simulink model "joint_impedance_control"  (R2025a)
settings: Solver=FixedStepDiscrete  StartTime=0.0  StopTime=inf  FixedStep=0.001  RelTol=1e-3
PreLoadFcn:
  | frs = FrankaRobotSettings;
libraries: franka_simulink x1
settings Model: SimulationMode=external  ExtModeTrigDuration=10000  Creator=vasi_ko  LastModifiedBy=kvasios
settings SolverCC: ConcurrentTasks=on  AlgebraicLoopSolver=TrustRegion
settings DataIOCC: LimitDataPoints=on  SaveFormat=Array  ReturnWorkspaceOutputs=off
settings OptimizationCC: EnhancedBackFolding=on  PassReuseOutputArgsThreshold=0.0  OptimizeBlockOrder=speed  DifferentSizesBufferReuse=on  OptimizationCustomize=off
settings DebuggingCC: SolverPrmCheckMsg=warning  ParameterTunabilityLossMsg=error  UnconnectedInputMsg=warning  UnconnectedOutputMsg=warning  UnconnectedLineMsg=warning  SFUnexpectedBacktrackingDiag=warning  SFNoUnconditionalDefaultTransitionDiag=warning  SFExecutionAtInitializationDiag=none  ArithmeticOperatorsInVariantConditions=warning
settings HardwareCC: ProdBitPerLong=64.0  ProdHWDeviceType=Intel->x86-64 (Linux 64)
settings ModelReferenceCC: EnableRefExpFcnMdlSchedulingChecks=on  PropagateSignalLabelsOutOfModel=off
settings SFSimCC: SimUseLocalCustomCode=off  MATLABDynamicMemAlloc=off  CustomCodeUndefinedFunction=UseInterfaceOnly  SimTargetLang=C++  SimDLTargetLibrary=mkl-dnn
settings RTWCC: HardwareBoard=Generic Linux AMD64 Board  RTWUseLocalCustomCode=off  BuildConfiguration=Faster Runs  TargetLang=C++  GPUComputeCapability=3.5  DLArmComputeVersion=19.05
settings CodeAppCC: ForceParamTrailComments=on  OperatorAnnotations=on
settings GRTTargetCC: ExtMode=on  ExtModeStaticAlloc=on  ExtModeMexFile=ext_xcp  ExtModeIntrfLevel=Level2 - Open  TargetLangStandard=C++14 (ISO)
settings ConfigComp: CovMetricSettings=dw  CovSaveCumulativeToWorkspaceVar=on  CovSaveSingleToWorkspaceVar=on  CovExternalEMLEnable=off  CovSFcnEnable=off

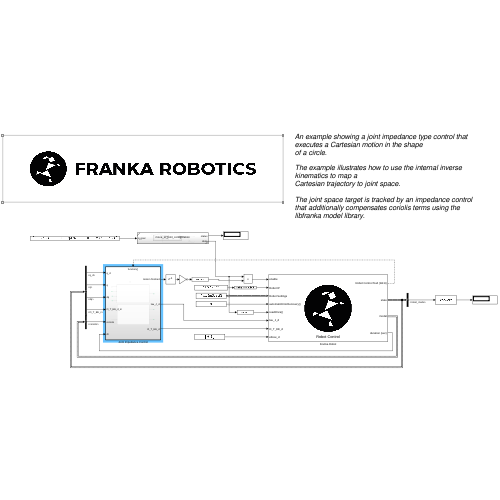
[thumbnail: Simulink's stored preview of the top-level diagram]
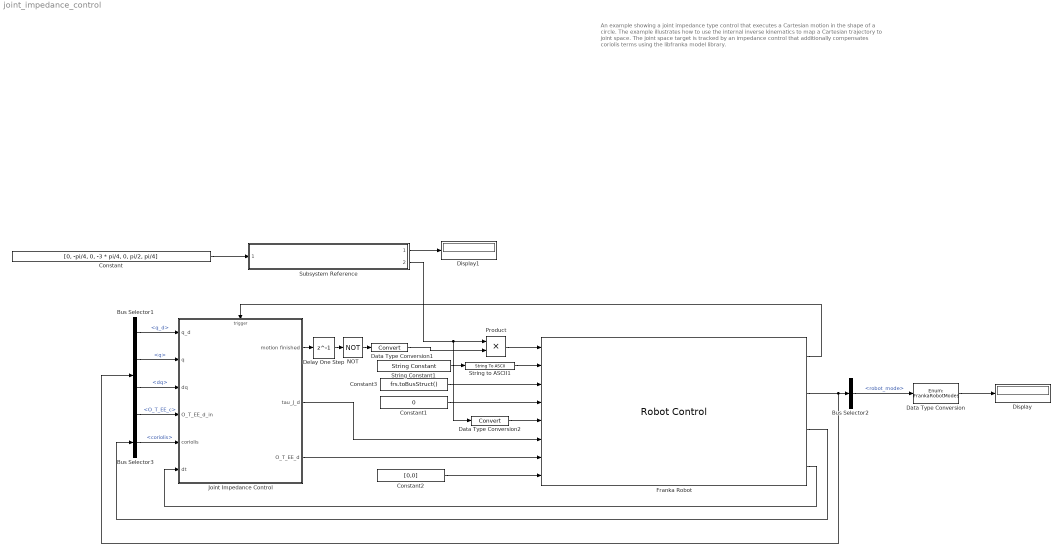
== system joint_impedance_control ==
  note: An example showing a joint impedance type control that executes a Cartesian motion in the shape
      | of a circle.
      |
      | The example illustrates how to use the internal inverse kinematics to map a
      | Cartesian trajectory to joint space.
      |
      | The joint space target is tracked by an impedance control
      | that additionally compensates coriolis terms using the libfranka model library.
  Bus Selector1 : BusSelector  OutputSignals=q_d,q,dq,O_T_EE_c
  Bus Selector2 : BusSelector  OutputSignals=robot_mode
  Bus Selector3 : BusSelector  OutputSignals=coriolis
  Constant : Constant  Value=[0, -pi/4, 0, -3 * pi/4, 0, pi/2, pi/4]
  Constant1 : Constant  Value=0  OutDataTypeStr=Inherit: Inherit via back propagation
  Constant2 : Constant  Value=[0,0]  OutDataTypeStr=Inherit: Inherit via back propagation
  Constant3 : Constant  Value=frs.toBusStruct()  OutDataTypeStr=Bus: FrankaRobotSettingsBus
  Data Type Conversion : DataTypeConversion  OutDataTypeStr=Enum: FrankaRobotModes  SaturateOnIntegerOverflow=off  RndMeth=Floor
  Data Type Conversion1 : DataTypeConversion  SaturateOnIntegerOverflow=off  RndMeth=Floor
  Data Type Conversion2 : DataTypeConversion  SaturateOnIntegerOverflow=off  RndMeth=Floor
  Delay One Step : Delay  DelayLength=1
  Display : Display
  Display1 : Display
  Franka Robot : franka_simulink/Robot Control  control_mode=Torques + Cartesian Pose
      settings: SourceProductName=Franka Robotics Simulink Support Package
  Joint Impedance Control : Subsystem  TreatAsAtomicUnit=on
      settings: RTWSystemCode=Nonreusable function
  NOT : Logic  Operator=NOT  IconShape=distinctive  AllPortsSameDT=off  OutDataTypeStr=boolean
  Product : Product
  String Constant1 : StringConstant  String="\"172.16.0.2\""
  String to ASCII1 : StringToASCII  OutputVectorSize=16
  Subsystem Reference : Subsystem  ReferencedSubsystem=move_to_joint_configuration
  wires:
  Constant/1 -> Subsystem Reference/1
  Bus Selector2/1 -> Data Type Conversion/1  "<robot_mode>"
  Constant3/1 -> Franka Robot/3
  Franka Robot/4 -> Joint Impedance Control/6(dt)
  Joint Impedance Control/1(motion finished) -> Delay One Step/1
  Constant1/1 -> Franka Robot/4
  NOT/1 -> Data Type Conversion1/1
  Data Type Conversion1/1 -> Product/2
  Franka Robot/3 -> Bus Selector3/1
  Subsystem Reference/2 -> Product/1, Data Type Conversion2/1
  Franka Robot/1 -> Joint Impedance Control/Trigger
  Delay One Step/1 -> NOT/1
  Data Type Conversion/1 -> Display/1
  Franka Robot/2 -> Bus Selector1/1, Bus Selector2/1
  String Constant1/1 -> String to ASCII1/1
  Subsystem Reference/1 -> Display1/1
  String to ASCII1/1 -> Franka Robot/2
  Constant2/1 -> Franka Robot/8
  Joint Impedance Control/3(O_T_EE_d) -> Franka Robot/7
  Joint Impedance Control/2(tau_J_d) -> Franka Robot/6
  Bus Selector3/1 -> Joint Impedance Control/5(coriolis)  "<coriolis>"
  Bus Selector1/1 -> Joint Impedance Control/1(q_d)  "<q_d>"
  Bus Selector1/2 -> Joint Impedance Control/2(q)  "<q>"
  Bus Selector1/3 -> Joint Impedance Control/3(dq)  "<dq>"
  Product/1 -> Franka Robot/1
  Data Type Conversion2/1 -> Franka Robot/5
  Bus Selector1/4 -> Joint Impedance Control/4(O_T_EE_d_in)  "<O_T_EE_c>"

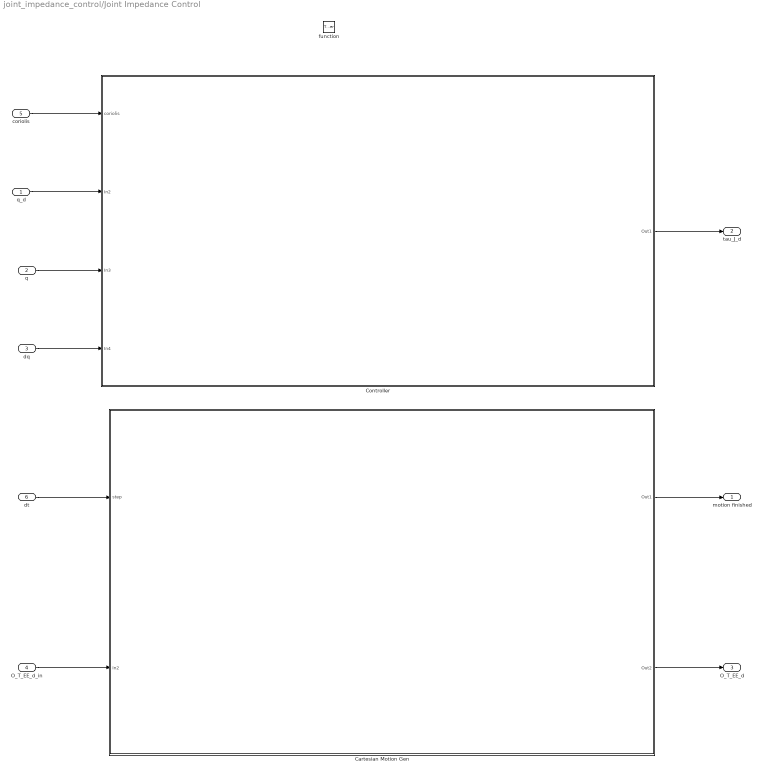
== system joint_impedance_control/Joint Impedance Control ==
  q_d : Inport
  q : Inport  Port=2
  dq : Inport  Port=3
  O_T_EE_d_in : Inport  Port=4
  coriolis : Inport  Port=5
  dt : Inport  Port=6
  function : TriggerPort  TriggerType=function-call  VariantControl=(inherit)
  Cartesian Motion Gen : Subsystem  TreatAsAtomicUnit=on
  Controller : Subsystem  TreatAsAtomicUnit=on
  motion finished : Outport  VectorParamsAs1DForOutWhenUnconnected=off
  tau_J_d : Outport  Port=2  VectorParamsAs1DForOutWhenUnconnected=off
  O_T_EE_d : Outport  Port=3  VectorParamsAs1DForOutWhenUnconnected=off
  wires:
  coriolis/1 -> Controller/1(coriolis)
  q_d/1 -> Controller/2(In2)
  q/1 -> Controller/3(In3)
  dq/1 -> Controller/4(In4)
  Controller/1(Out1) -> tau_J_d/1
  dt/1 -> Cartesian Motion Gen/1(step)
  O_T_EE_d_in/1 -> Cartesian Motion Gen/2(In2)
  Cartesian Motion Gen/1(Out1) -> motion finished/1
  Cartesian Motion Gen/2(Out2) -> O_T_EE_d/1

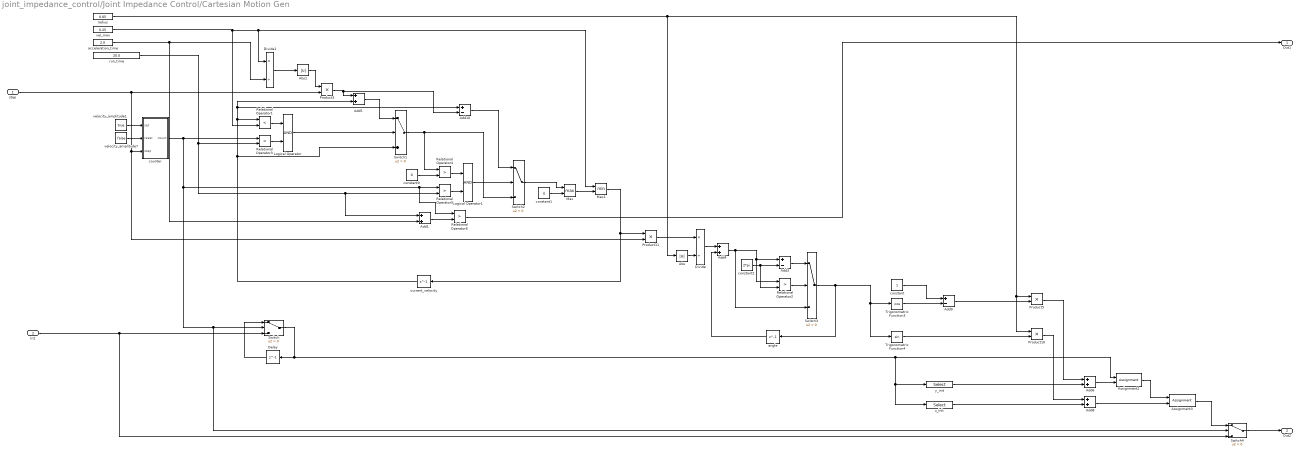
== system joint_impedance_control/Joint Impedance Control/Cartesian Motion Gen ==
  step : Inport
  In2 : Inport  Port=2
  Abs : Abs  SaturateOnIntegerOverflow=off
  Abs1 : Abs  SaturateOnIntegerOverflow=off
  Add{1,4..6,8} (5 alike) : Sum
  Add10 : Sum  Inputs=+-
  Add3 : Sum  Inputs=+-
  Add9 : Sum  Inputs=+-
  Assignment2 : Assignment  NumberOfDimensions=2  DiagnosticForDimensions=Warning  IndexOptions=Index vector (dialog),Index vector (dialog)  Indices=2,4  OutputSizes=1,1
  Assignment3 : Assignment  NumberOfDimensions=2  DiagnosticForDimensions=Warning  IndexOptions=Index vector (dialog),Index vector (dialog)  Indices=3,4  OutputSizes=1,1
  Delay : Delay  DelayLength=1
  Divide : Product  Inputs=*/
  Divide1 : Product  Inputs=*/
  Logical Operator : Logic  AllPortsSameDT=off  OutDataTypeStr=boolean
  Logical Operator1 : Logic  AllPortsSameDT=off  OutDataTypeStr=boolean
  Max : MinMax  Function=max  Inputs=2
  Max1 : MinMax  Inputs=2
  Product{3,5,10..11} (4 alike) : Product
  Relational Operator1 : RelationalOperator  Operator=<  OutDataTypeStr=boolean  InputSameDT=off
  Relational Operator{2,4..6} (4 alike) : RelationalOperator  Operator=>  OutDataTypeStr=boolean  InputSameDT=off
  Relational Operator3 : RelationalOperator  Operator=<  OutDataTypeStr=boolean  InputSameDT=off
  Switch{,1..4} (5 alike) : Switch  Criteria=u2 > Threshold  SaturateOnIntegerOverflow=off  InputSameDT=off
  Trigonometric Function3 : Trigonometry  Operator=cos  NumberOfIterations=50
  Trigonometric Function4 : Trigonometry  NumberOfIterations=50
  acceleration_time : Constant  Value=2.0  VectorParams1D=off
  angle : Delay  DelayLength=1  InitialCondition=0
  constant : Constant  VectorParams1D=off
  constant0 : Constant  Value=0  VectorParams1D=off
  constant1 : Constant  Value=0  VectorParams1D=off
  constant2 : Constant  Value=2*pi  VectorParams1D=off
  counter : Subsystem
  current_velocity : Delay  DelayLength=1  InitialCondition=0
  radius : Constant  Value=0.05  VectorParams1D=off
  run_time : Constant  Value=20.0  VectorParams1D=off
  vel_max : Constant  Value=0.25  VectorParams1D=off
  velocity_amplitude1 : Constant  Value=true  VectorParams1D=off
  velocity_amplitude7 : Constant  Value=false  VectorParams1D=off
  y_init : Selector  NumberOfDimensions=2  InputPortWidth=16  IndexOptions=Index vector (dialog),Index vector (dialog)  Indices=2,4  OutputSizes=1,1
  z_init : Selector  NumberOfDimensions=2  InputPortWidth=16  IndexOptions=Index vector (dialog),Index vector (dialog)  Indices=3,4  OutputSizes=1,1
  Out1 : Outport
  Out2 : Outport  Port=2
  wires:
  Add8/1 -> Assignment3/2
  Abs1/1 -> Product3/1
  Switch2/1 -> Max/1
  Divide1/1 -> Abs1/1
  Max/1 -> Max1/2
  Trigonometric Function3/1 -> Add9/2
  acceleration_time/1 -> Add1/2, Divide1/2
  Divide/1 -> Add4/1
  Trigonometric Function4/1 -> Product10/2
  z_init/1 -> Add8/2
  Relational Operator3/1 -> Logical Operator/2
  Add9/1 -> Product5/2
  counter/1(count) -> Switch4/2, Switch/2, Relational Operator6/1, Relational Operator5/1, Relational Operator3/1
  Logical Operator1/1 -> Switch2/2
  In2/1 -> Switch4/3, Switch/3
  Switch1/1 -> Relational Operator4/1, Switch2/3
  angle/1 -> Add4/2
  velocity_amplitude7/1 -> counter/2(reset)
  Product11/1 -> Divide/1
  constant1/1 -> Max/2
  Product3/1 -> Add10/2, Add5/1
  vel_max/1 -> Max1/1, Divide1/1, Relational Operator1/2
  Relational Operator2/1 -> Switch3/2
  run_time/1 -> Add1/1, Relational Operator5/2, Relational Operator3/2
  velocity_amplitude1/1 -> counter/1(set)
  y_init/1 -> Add6/2
  Max1/1 -> current_velocity/1, Product11/1
  Add3/1 -> Switch3/1
  step/1 -> Product11/2, counter/3(step), Product3/2
  Switch4/1 -> Out2/1
  Assignment3/1 -> Switch4/1
  Add4/1 -> Relational Operator2/1, Add3/1, Switch3/3
  constant2/1 -> Relational Operator2/2, Add3/2
  Switch3/1 -> angle/1, Trigonometric Function4/1, Trigonometric Function3/1
  Product10/1 -> Add8/1
  Add6/1 -> Assignment2/2
  radius/1 -> Product10/1, Product5/1, Abs/1
  Product5/1 -> Add6/1
  Add5/1 -> Switch1/1
  constant0/1 -> Relational Operator4/2
  Relational Operator1/1 -> Logical Operator/1
  Add10/1 -> Switch2/1
  Delay/1 -> Switch/1
  Logical Operator/1 -> Switch1/2
  Assignment2/1 -> Assignment3/1
  Abs/1 -> Divide/2
  Switch/1 -> z_init/1, y_init/1, Assignment2/1, Delay/1
  constant/1 -> Add9/1
  current_velocity/1 -> Switch1/3, Add10/1, Add5/2, Relational Operator1/1
  Relational Operator5/1 -> Logical Operator1/2
  Relational Operator4/1 -> Logical Operator1/1
  Add1/1 -> Relational Operator6/2
  Relational Operator6/1 -> Out1/1

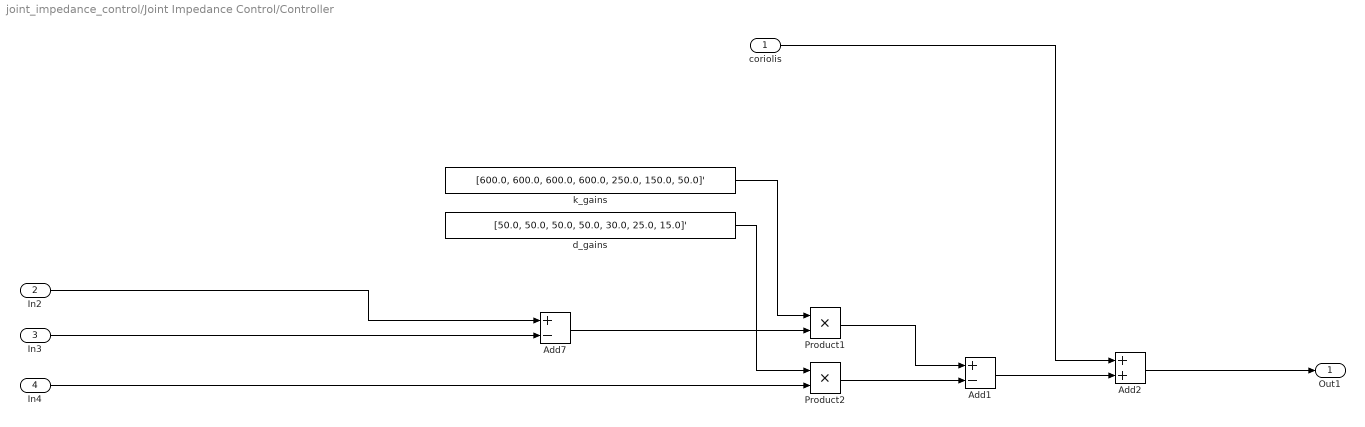
== system joint_impedance_control/Joint Impedance Control/Controller ==
  coriolis : Inport
  In2 : Inport  Port=2
  In3 : Inport  Port=3
  In4 : Inport  Port=4
  Add1 : Sum  Inputs=+-
  Add2 : Sum
  Add7 : Sum  Inputs=+-
  Product1 : Product
  Product2 : Product
  d_gains : Constant  Value=[50.0, 50.0, 50.0, 50.0, 30.0, 25.0, 15.0]'  VectorParams1D=off
  k_gains : Constant  Value=[600.0, 600.0, 600.0, 600.0, 250.0, 150.0, 50.0]'  VectorParams1D=off
  Out1 : Outport
  wires:
  Product2/1 -> Add1/2
  Add1/1 -> Add2/2
  Add7/1 -> Product1/2
  In4/1 -> Product2/2
  k_gains/1 -> Product1/1
  d_gains/1 -> Product2/1
  coriolis/1 -> Add2/1
  In2/1 -> Add7/1
  Product1/1 -> Add1/1
  Add2/1 -> Out1/1
  In3/1 -> Add7/2

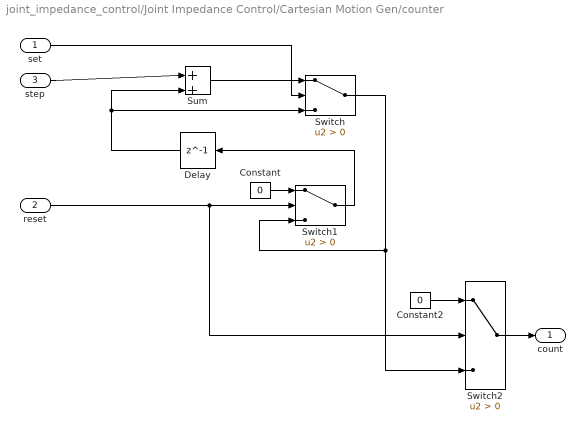
== system joint_impedance_control/Joint Impedance Control/Cartesian Motion Gen/counter ==
  set : Inport  OutDataTypeStr=boolean
  reset : Inport  Port=2  OutDataTypeStr=boolean
  step : Inport  Port=3  OutDataTypeStr=double
  Constant : Constant  Value=0  OutDataTypeStr=double
  Constant2 : Constant  Value=0  OutDataTypeStr=double
  Delay : Delay  DelayLength=1  InitialCondition=0
  Sum : Sum  Inputs=|++
  Switch : Switch  Criteria=u2 > Threshold  SaturateOnIntegerOverflow=off  InputSameDT=off
  Switch1 : Switch  Criteria=u2 > Threshold  OutDataTypeStr=double  SaturateOnIntegerOverflow=off  InputSameDT=off
  Switch2 : Switch  Criteria=u2 > Threshold  OutDataTypeStr=double  SaturateOnIntegerOverflow=off  InputSameDT=off
  count : Outport  OutDataTypeStr=double  VectorParamsAs1DForOutWhenUnconnected=off
  wires:
  Switch1/1 -> Delay/1
  Constant/1 -> Switch1/1
  reset/1 -> Switch2/2, Switch1/2
  Delay/1 -> Switch/3, Sum/2
  step/1 -> Sum/1
  Switch/1 -> Switch2/3, Switch1/3
  set/1 -> Switch/2
  Sum/1 -> Switch/1
  Constant2/1 -> Switch2/1
  Switch2/1 -> count/1
